simulink library "EmE_MBD_Blockset"  (R2018a)
settings: Solver=ode1  StartTime=0.0  StopTime=Inf  FixedStep=0.001  RelTol=1e-3  EnableMultiTasking=on
PostLoadFcn:
  | , if any(exist('dsrtsu_mdlpostloadfcn', 'file') == [2, 3, 6]), try dsrtsu_mdlpostloadfcn('Execute', bdroot); catch fprintf('Error in PostLoadFcn (dsrtsu_mdlpostloadfcn) for model "%s":\n %s\n', bdroot, lasterr); end, end,
undefined symbols (not defined in the file or in its folder): ENUM_TSC1_CONTROL_PURPOSE_T, gcbh, GLB_SWITCH_T
libraries: simulink x237, $bdroot x115, simulink_need_slupdate x26, MotoHawk_lib x13, simulink_extras x3
(part 2 of 11)

== system EmE_MBD_Blockset/Math Operators ==
  Abs : Abs  mask(Absolute value (EmE)){SaturateOnIntegerOverflow=off}
      mask prompts: SaturateOnIntegerOverflow "Simulink:blkprm_prompts:AllBlksSaturate"
      mask help: Outputs the absolute value of the input.
      mask TypeOptions SaturateOnIntegerOverflow: SaturateOnIntegerOverflow
      mask DialogControl SaturateOnIntegerOverflow Prompt: Saturate on integer overflow
  Add : Sum  InputSameDT=on
  Convert_polar_coordinates_to_rectangular_coordinates : Subsystem
  Convert_rectangular_coordinates_to_polar_coordinates : Subsystem
  Convert_time : Subsystem  mask(Convert units of time (EmE)){cvt_time_from=hr, cvt_time_to=min, sat_on_int_overflow=off}
      mask prompts: cvt_time_from "Convert time from"; cvt_time_to "Convert time to"; sat_on_int_overflow "Saturate on integer overflow"
      mask help:
      | Converts one unit of time to another.  Available time units are:
      | - microsecond (usec)
      | - millisecond (msec)
      | - second (sec)
      | - minute (min)
      | - hour (hr)
      | - day (day)
      | - year (yr)
      mask init:
      | constant = [get_param(gcbh,'Parent'),'/',get_param(gcbh,'name'),'/Constant'];
      | product1 = [get_param(gcbh,'Parent'),'/',get_param(gcbh,'name'),'/Product1'];
      | 
      | time_labels = ...
      |     { 'usec' 
      |       'msec' 
      |       'sec' 
      |       'min'
      |       'hr' 
      |       'day' 
      |       'yr' };
      | conversions_time = ...
      |     { '1'
      |       '1000'
      |       '1000'
      |       '60'
      |       '60'
      |       '24'
      |       '365'};
      | 
      | from_nr = find(strcmp(time_labels, cvt_time_from));
      | to_nr   = find(strcmp(time_labels, cvt_time_to));
      | 
      | conversion_factor = '1';
      | if ( from_nr < to_nr )
      |     for i = from_nr+1:to_nr
      |         conversion_factor = [conversion_factor, '/', conversions_time{i}];
      |     end
      | elseif ( from_nr > to_nr )
      |     for i = to_nr+1:from_nr
      |         conversion_factor = [conversion_factor, '*', conversions_time{i}];
      |     end
      | end
      | set_param(constant, 'Value', conversion_factor);
      | set_param(product1, 'SaturateOnIntegerOverflow', sat_on_int_overflow);
      mask TypeOptions cvt_time_from: usec | msec | sec | min | hr | day | yr
      mask TypeOptions cvt_time_to: usec | msec | sec | min | hr | day | yr
      mask Display: disp([cvt_time_from ' to ' cvt_time_to])
  Decrement Real World : simulink/Additional Math & Discrete/Additional Math: Increment - Decrement/Decrement Real World
      settings: SourceProductName=Simulink  SourceProductBaseCode=SL
  Divide : Product  Inputs=*/  InputSameDT=on
  Engineering_unit_conversion : Subsystem  mask(Convert engineering units (EmE)){eng_unit_type=torque, eng_unit_in=Nm, eng_unit_out=lbf-ft, sat_on_int_overflow=off}
      mask prompts: eng_unit_type "Unit type:"; eng_unit_in "Convert from:"; eng_unit_out "Convert to:"; sat_on_int_overflow "Saturate on integer overflow"
      mask help: Converts one engineering unit to another.
      mask init:
      | % https://www.mathworks.com/matlabcentral/fileexchange/3181-unit-conversion
      | unit_labels = {'accel','angle','area','density','energy','flow','flow_num','force','freq','fuel_econ','inertia','length','velocity','mass','power','pressure','spec_heat','temp','torque','kin_vis','vol'};
      | switch eng_unit_type,
      |     case 'accel',
      |         eng_unit_opts = {'cm/s2','ft/s2','g','m/s2','mi/hr-s','mm/s2'};
      |     case 'angle',
      |         eng_unit_opts = {'cycle','rad','deg','min','sec'};
      |     case 'area',
      |         eng_unit_opts = {'km2','hectare','m2','cm2','mm2','mile2','acre','ft2','in2'};
      |     case 'density',
      |         eng_unit_opts = {'tonne/m3','kg/m3','sg','lb/in3','lb/ft3','lb/igal','lb/usgal','slug/ft3'};
      |     case 'energy',
      |         eng_unit_opts = {'MJ','J','kWh','cal','chu','therm','btu','ft-lbf','hp-s'};
      |     case 'flow',
      |         eng_unit_opts = {'m3/s','liter/s','cc/s','in3/s','gal/hr','kg/s','lb/s','lb/hr','ft3/min'};
      |     case 'flow_num',
      |         eng_unit_opts = {'cc/s/sq(kPa)','ss/s/sq(bar)','gph/sq(psi)','in3/s/sq(psi)'};
      |     case 'force',
      |         eng_unit_opts = {'bar-m2','kN','N','kPa-mm2','dyne','kgf','tonf','lbf','pdl'};
      |     case 'freq',
      |         eng_unit_opts = {'1/ms','hz','rad/s','deg/s','rpm','1/hour','1/day'};
      |     case 'fuel_econ',
      |         eng_unit_opts = {'100km/l','km/l','m/l','mi/igal','mi/usgal'};
      |     case 'inertia',
      |         eng_unit_opts = {'kg-m2','lb-ft2','lb-in2'};
      |     case 'length',
      |         eng_unit_opts = {'km','m','cm','mm','n-mile','mile','yard','ft','in'};
      |     case 'velocity',
      |         eng_unit_opts = {'km/s','km/hr','m/s','m/min','m/hr','knot','mph','ft/s','ft/hr'};
      |     case 'mass',
      |         eng_unit_opts = {'tonne','kg','g','ton','slug','stone','lb','oz','dr'};
      |     case 'power',
      |         eng_unit_opts = {'kw','w','chu/s','btu/s','btu/hr','ft-lbf/s','ps','hp'};
      |     case 'pressure',
      |         eng_unit_opts = {'MPa','bar','kPa','Pa','atm','ton/in2','psi','mmHg'};
      |     case 'spec_heat',
      |         eng_unit_opts = {'kJ/kg-K','J/kg-K','chu/lb-K','btu/lb-R','hp-s/lb-K','ft-lbf/lb-R'};
      |     case 'temp',
      |         eng_unit_opts = {'K','C','R','F'};
      |     case 'torque',
      |         eng_unit_opts = {'Nm','lbf-ft','lbf-in'};
      |     case 'kin_vis',
      |         eng_unit_opts = {'m2/s','cm2/s','cStoke','ft2/s','in2/s'};
      |     case 'vol',
      |         eng_unit_opts = {'m3','liter','cm3','mm3','ft3','in3','igal','pint','usgal'};
      | end;
      | % set table parameters
      | unit_type_idx = [];
      | unit_in_type_idx = [];
      | unit_out_type_idx = [];
      | user_sg=1; % specific gravity value used... need to add to dialog?
      | try
      |     unit_type_idx = find(strcmpi(unit_labels, eng_unit_type));
      |     unit_in_type_idx = find(strcmpi(eng_unit_opts, eng_unit_in));
      |     unit_out_type_idx = find(strcmpi(eng_unit_opts, eng_unit_out));
      | catch
      | end;
      | if (~isempty(unit_type_idx) && ~isempty(unit_in_type_idx) && ~isempty(unit_out_type_idx)),
      |     % Set output size
      |     opsiz=[1,1];
      |     oplen=prod(opsiz);
      |     
      |     % Define basic numbers
      |     yd=1/0.9144; yd2=yd^2; yd3=yd*yd2; mi=1760; acr=4840; gal=1/4.546092; usgl=231;
      |     lb=1/0.45359237; ton=2240; g=9.80665; atm=101.325; hg=750.0616827e-5;
      |     ps=1/75; hp=550; cal=0.238846; chu=1/1899.1005354; k2r=1.8; abz=273.15;
      |     sg=1;
      |     
      |     % For future development - if required
      |     % angstrom=1e-10m; rod=5.5yard; chain=22yard; furlong=10chain; fathom=2yard;
      |     % short_ton=2000 lb; cwt=112 lb; lb=7000grain; metric_carat=0.2g;
      |     % chaldron=36bushel; barrel=36gal bushel=8gal; peck=2gal; quart=2pint; pint=4gill; gill=5fl.oz; fl.oz=8fl.drachm
      |     
      |     fact = [...
      |         1,0.0328083,0.0010197,0.01,0.0223692,10,0,0,0;...                                               % accel
      |         1/2,pi,180,180*60,180*3600,0,0,0,0;...                                                          % angle
      |         1e-6,1e-4,1,1e4,1e6,yd2/mi^2,yd2/acr,9*yd2,1296*yd2;...                                         % area
      |         1e-3,1,1e-3,lb/(46656*yd3),lb/(27*yd3),lb/(1e3*gal),lb*usgl/(46656*yd3),lb/(81*yd2^2*g),0;...   % density
      |         1e-6,1,1e-6/3.6,cal,chu,chu*k2r*1e-5,chu*k2r,3*yd*lb/g,3*yd*lb/g/hp;...                         % energy
      |         1e-6,1e-3,1,0.046656*yd3,gal*3.6,sg*1e-3,lb*sg*1e-3,lb*sg*1e-1*36,0.00211888;...                % flow
      |         1,10,gal*yd*12.96*sqrt(0.1*g/lb),(0.1296*yd2)^2*sqrt(10*g/lb),0,0,0,0,0;...                     % flow_num
      |         1e-5,1e-3,1,1e3,1e5,1/g,lb/(g*ton),lb/g,lb*yd*3;...                                             % force
      |         1e-3,1,2*pi,360,60,3600,86400,0,0;...                                                           % freq
      |         1e-5,1e-3,1,yd/(mi*gal),yd*usgl/(mi*yd3*46.656),0,0,0,0;...                                     % fuel_econ
      |         1,lb*9*yd2,lb*1296*yd2,0,0,0,0,0,0;...                                                          % inertia
      |         1e-3,1,100,1000,1/1852,yd/mi,yd,3*yd,36*yd;...                                                  % length
      |         1e-3,3.6,1,60,3600,3600/1852,yd*3600/mi,3*yd,3*yd*3600;...                                      % velocity
      |         1e-3,1,1000,lb/ton,lb/(yd*3*g),lb/14,lb,lb*16,lb*16^2;...                                       % mass
      |         1e-3,1,chu,chu*k2r,chu*k2r*3600,3*yd*lb/g,ps/g,3*yd*lb/g/hp,0;...                               % power
      |         1e-6,1e-5,1e-3,1,1e-3/atm,lb/(1296*ton*g*yd2),lb/(1296*g*yd2),hg,0;...                          % pressure
      |         1e-3,1,chu/lb,chu/lb,3*yd/(g*hp),3*yd/g/k2r,0,0,0;...                                           % spec_heat
      |         1,1,k2r,k2r,0,0,0,0,0;...                                                                       % temp
      |         1,0.737561,8.85075,0,0,0,0,0,0;...                                                              % torque
      |         1,1e4,1e6,9*yd2,1296*yd2,0,0,0,0;...                                                            % kin_vis
      |         1,1e3,1e6,1e9,27*yd3,27*yd3*1728,1e3*gal,gal*8000,yd3*46656/usgl;...                            % vol
      |         ];
      |     off = [abz,0,abz,32/k2r,0,0,0,0,0];                                                                 % temp
      |     
      |     % Set factor
      |     % sub2ind indexes into a matrix; matrix(a,b) is a matrix if both a & b are vectors
      |     ind=sub2ind( size(fact), ones(oplen,1).*unit_type_idx(:), ones(oplen,1).*unit_in_type_idx(:) );
      |     in_fact=fact(ind);
      |     ind=sub2ind( size(fact), ones(oplen,1).*unit_type_idx(:), ones(oplen,1).*unit_out_type_idx(:) );
      |     out_fact=fact(ind);
      |     
      |     % Set offset - apply if unit_type_idx==18(temp), else 0
      |     in_off=off(unit_in_type_idx(:))'.*(unit_type_idx(:)==18);
      |     out_off=off(unit_out_type_idx(:))'.*(unit_type_idx(:)==18);
      |     
      |     % Previous un-vectorised code:-
      |     % If user chose Qflow & Mflow use sg - sg defaults 1, keep here in case it's changed
      |     %if unit_type_idx==5 & ((unitinput>5) ~= (unitoutput>5))
      |     %  if unitinput>5 then
      |     %     in_fact = in_fact(:) .* user_sg(:)/sg;
      |     %  else
      |     %     out_fact = out_fact(:) .* user_sg(:)/sg;
      |     %  end;
      |     %end;
      |     % This sg thing adds a complication for vector/matrix arithmetic:
      |     flow_conv=(unit_type_idx(:)==6 & ((unit_in_type_idx(:)>6) ~= (unit_out_type_idx(:)>6))); % vector of whether sg is needed
      |     ip_gt_6=(unit_in_type_idx(:)>6)*2-1;  % vector of 1 or -1 s : 1->multiply; (-1)->divide
      |     in_fact = in_fact(:) .* ((user_sg(:)/sg) .^ flow_conv).^ip_gt_6;
      |     
      |     % Set factor & offset
      |     factor_u=out_fact(:)./in_fact(:);
      |     offset_u=(out_off(:)-in_off(:)).*out_fact(:);
      |     
      |     % Reshape to match unitinput matrix size
      |     factor_u=reshape(factor_u,opsiz);
      |     offset_u=reshape(offset_u,opsiz);
      | end;
      | % assign values in simulink block
      | gain_value = [get_param(gcbh,'Parent'),'/',get_param(gcbh,'name'),'/Gain_value'];
      | offset_value = [get_param(gcbh,'Parent'),'/',get_param(gcbh,'name'),'/Offset_value'];
      | set_param(gain_value, 'Value', num2str(factor_u));
      | set_param(offset_value, 'Value', num2str(offset_u));
      mask TypeOptions eng_unit_type: accel | angle | area | density | energy | flow | flow_num | force | freq | fuel_econ | inertia | length | velocity | mass | power | pressure | spec_heat | temp | torque | kin_vis | vol
      mask Callback eng_unit_type:
      | % https://www.mathworks.com/matlabcentral/answers/82930-dynamically-populating-mask-parameter-popup-list
      | % get the unit type selected
      | eng_unit_type_gcbh = get(gcbh);
      | eng_unit_type = eng_unit_type_gcbh.eng_unit_type;
      | % begin to set the 'from' and 'to' unit type drop down menus
      | maskstyles = get_param(gcb, 'MaskStyles');
      | switch eng_unit_type,
      |     case 'accel',
      |         eng_unit_opts = 'popup(cm/s2|ft/s2|g|m/s2|mi/hr-s|mm/s2)';
      |     case 'angle',
      |         eng_unit_opts = 'popup(cycle|rad|deg|min|sec)';
      |     case 'area',
      |         eng_unit_opts = 'popup(km2|hectare|m2|cm2|mm2|mile2|acre|ft2|in2)';
      |     case 'density',
      |         eng_unit_opts = 'popup(tonne/m3|kg/m3|sg|lb/in3|lb/ft3|lb/igal|lb/usgal|slug/ft3)';
      |     case 'energy',
      |         eng_unit_opts = 'popup(MJ|J|kWh|cal|chu|therm|btu|ft-lbf|hp-s)';
      |     case 'flow',
      |         eng_unit_opts = 'popup(m3/s|liter/s|cc/s|in3/s|gal/hr|kg/s|lb/s|lb/hr|ft3/min)';
      |     case 'flow_num',
      |         eng_unit_opts = 'popup(cc/s/sq(kPa)|ss/s/sq(bar)|gph/sq(psi)|in3/s/sq(psi))';
      |     case 'force',
      |         eng_unit_opts = 'popup(bar-m2|kN|N|kPa-mm2|dyne|kgf|tonf|lbf|pdl)';
      |     case 'freq',
      |         eng_unit_opts = 'popup(1/ms|hz|rad/s|deg/s|rpm|1/hour|1/day)';
      |     case 'fuel_econ',
      |         eng_unit_opts = 'popup(100km/l|km/l|m/l|mi/igal|mi/usgal)';
      |     case 'inertia',
      |         eng_unit_opts = 'popup(kg-m2|lb-ft2|lb-in2)';
      |     case 'length',
      |         eng_unit_opts = 'popup(km|m|cm|mm|n-mile|mile|yard|ft|in)';
      |     case 'velocity',
      |         eng_unit_opts = 'popup(km/s|km/hr|m/s|m/min|m/hr|knot|mph|ft/s|ft/hr)';
      |     case 'mass',
      |         eng_unit_opts = 'popup(tonne|kg|g|ton|slug|stone|lb|oz|dr)';
      |     case 'power',
      |         eng_unit_opts = 'popup(kw|w|chu/s|btu/s|btu/hr|ft-lbf/s|ps|hp)';
      |     case 'pressure',
      |         eng_unit_opts = 'popup(MPa|bar|kPa|Pa|atm|ton/in2|psi|mmHg)';
      |     case 'spec_heat',
      |         eng_unit_opts = 'popup(kJ/kg-K|J/kg-K|chu/lb-K|btu/lb-R|hp-s/lb-K|ft-lbf/lb-R)';
      |     case 'temp',
      |         eng_unit_opts = 'popup(K|C|R|F)';
      |     case 'torque',
      |         eng_unit_opts = 'popup(Nm|lbf-ft|lbf-in)';
      |     case 'kin_vis',
      |         eng_unit_opts = 'popup(m2/s|cm2/s|cStoke|ft2/s|in2/s)';
      |     case 'vol',
      |         eng_unit_opts = 'popup(m3|liter|cm3|mm3|ft3|in3|igal|pint|usgal)';
      | end;
      | 
      | % set the other drop down menu boxes with the selectable units
      | maskstyles{2} = eng_unit_opts;
      | maskstyles{3} = eng_unit_opts;
      | set_param(gcb, 'MaskStyles', maskstyles);
      mask TypeOptions eng_unit_in: Nm | lbf-ft | lbf-in
      mask TypeOptions eng_unit_out: Nm | lbf-ft | lbf-in
      mask Display:
      | % sprintf('%s/n%s to %s',[engunittype,engunitinput,engunitoutput])
      | disp([eng_unit_type '\n' eng_unit_in ' to ' eng_unit_out])
  Find Nonzero Elements : Find  NumberOfInputDimensions=3  IndexMode=Zero-based
  Gain : Gain
  Generic_linear_function : Subsystem  mask(Generic linear function (EmE)){}
      mask help: Linear interpolation function for x-y interpolation. Output is bound by Y1 and Y2 values.
      mask init:
      | X_1=0.37;
      | X_2=0.65;
      | Y_1=0.37;
      | Y_2=0.8;
      mask Display:
      | %AXIS
      |     plot([0.2 0.8]+0.15,[0.3 0.3]+0.1);
      |     plot([0.25 0.25]+0.15,[0.25 0.97]+0.1);
      |     text(0.38,1.05,'y')
      |     text(0.93,0.39,'x')
      | 
      | % GRAPH
      |     plot([X_1 X_2]+0.15,[Y_1 Y_2]+0.1)
      | 
      | % TEXT and LINES
      | %X_1
      |     plot([X_1,X_1]+0.15,[0.37 0.36]+0.1);
      |     plot([X_1,X_1]+0.15,[0.34 0.33]+0.07);
      |     plot([X_1,X_1]+0.15,[0.33 0.31]+0.1);
      |     text(0.49,0.33,sprintf('%s\n','X1'))
      | 
      | %X_2
      |     plot([Y_1 Y_1]+0.43,[0.25 0.28]+0.61);
      |     plot([Y_1 Y_1]+0.43,[0.22 0.19]+0.61);
      |     plot([Y_1 Y_1]+0.43,[0.16 0.13]+0.61);
      |     plot([Y_1 Y_1]+0.43,[0.10 0.07]+0.61);
      |     plot([Y_1 Y_1]+0.43,[0.04 0.01]+0.61);
      |     plot([Y_1 Y_1]+0.43,[-0.02 -0.05]+0.61);
      |     plot([Y_1 Y_1]+0.43,[-0.08 -0.11]+0.61);
      |     plot([Y_1 Y_1]+0.43,[-0.14 -0.17]+0.61);
      |     plot([Y_1 Y_1]+0.43,[-0.20 -0.21]+0.61);
      |     text(0.77,0.33,sprintf('%s\n','X2'))
      | 
      | %Y_1
      |     plot([0.3 0.42]+0.1,[Y_1 Y_1]+0.1);
      |     text(0.3,0.48,'Y1')
      | 
      | %Y_2
      |     plot([0.25 0.28]+0.15,[X_2 X_2]+0.25);
      |     plot([0.31 0.34]+0.15,[X_2 X_2]+0.25);
      |     plot([0.37 0.40]+0.15,[X_2 X_2]+0.25);
      |     plot([0.43 0.46]+0.15,[X_2 X_2]+0.25);
      |     plot([0.49 0.52]+0.15,[X_2 X_2]+0.25);
      |     plot([0.55 0.58]+0.15,[X_2 X_2]+0.25);
      |     plot([0.61 0.64]+0.15,[X_2 X_2]+0.25);
      |     plot([0.65 0.8]+0.15,[X_2 X_2]+0.25);
      |     text(0.3,Y_2+0.1,'Y2')
      | 
      | %Center pic
      | text(0.16,1.3,' ')
      | text(1.1,0.1,' ')
  Increment Real World : simulink/Additional Math & Discrete/Additional Math: Increment - Decrement/Increment Real World
      settings: SourceProductName=Simulink  SourceProductBaseCode=SL
  Math Function : Math  SaturateOnIntegerOverflow=on
  MinMax : MinMax  Inputs=2  InputSameDT=on
  MinMax Running Resettable : simulink/Math Operations/MinMax Running Resettable  Function=min  vinit=0
      settings: AttributesFormatString=IC: %<vinit>
  Min_max_index : Subsystem  mask(Min max index (EmE)){func=max, sat_on_int_overflow=off}
      mask prompts: func "Function:"; sat_on_int_overflow "Saturate on integer overflow"
      mask help:
      | Output min or max of the inputs as well as the index of the winning input.  The inputs are prioritized from top to bottom.
      | Input to the block must be a bus or a mux.
      mask init:
      | minmaxblk = [get_param(gcbh,'parent'),'/',get_param(gcbh,'name'),'/MinMax'];
      | set_param(minmaxblk,'Function',func);
      mask TypeOptions func: min | max
      mask Display:
      | disp(func);
      | port_label('output', 1, 'v');
      | port_label('output', 2, 'i');
  Normalize_on_min_max : Subsystem  mask(Normalize on min, max (EmE)){sel=Min}
      mask prompts: sel "Normalize on:"
      mask help: Normalize the input on the minimum or maximum boundary.
      mask init:
      | cpv = [get_param(gcbh,'parent'),'/',get_param(gcbh,'name'),'/Constant'];
      | if strcmp(sel,'Min'),
      |     set_param(cpv,'Value','true');
      | else,
      |     set_param(cpv,'Value','false');
      | end
      mask TypeOptions sel: Min | Max
      mask Display:
      | plot([0.1 0.1 0.8 0.8],[0.3 0.7 0.7 0.3])
      | plot([0.1 0.8],[0.3 0.3])
      | text( 0.15, 0.5, 'norm =')
      | plot([0.4 0.75],[0.5 0.5])
      | text( 0.43, 0.4, '(max - min)')
      | if (strcmpi(sel,'Min')),
      |     text( 0.45, 0.6, '(in - min)')
      | else,
      |     text( 0.45, 0.6, '(max - in)')
      | end;
  Product : Product  InputSameDT=on
  Rounding Function : Rounding  mask(Rounding function (EmE)){Operator=floor}
      mask prompts: Operator "Simulink:blkprm_prompts:RoundOperator"
      mask help: Apply rounding function to signal.
      mask TypeOptions Operator: Operator
      mask DialogControl Operator Prompt: Function:
  Slew : Subsystem  mask(Slew (EmE)){}
      mask help:
      | Limits the maximum increase rate by 'Inc' and the maximum decrease rate by 'Dec'.
      | If In > Out, then Out is increased by Inc*dT every time step until Out = In.
      | If In < Out, then Out is decreased by Dec*dT every time step until Out = In.
      mask Display:
      | plot([0.1 1],[0.5 0.96])
      | plot([0.1 1],[0.5 0.04])
      | plot([0.1 0.7],[0.5 0.5])
      | plot([0.65 0.7],[0.55 0.5])
      | plot([0.65 0.7],[0.45 0.5])
      | 
      | plot([0 0.22],[0.8 0.58])
      | plot([0 0.22],[0.2 0.42])
      | plot([0.1 0.42],[1 0.68])
      | plot([0.1 0.42],[0 0.32])
      | plot([0.4 0.62],[1 0.78])
      | plot([0.4 0.62],[0 0.22])
      | plot([0.7 0.81],[1 0.88])
      | plot([0.7 0.81],[0 0.12])
  Slew_at_event : Subsystem  mask(Slew at event (EmE)){}
      mask help:
      | Performs a trigger-based slew that is initialized with value Init and slews towards In at a linear rate defined by Inc and Dec.
      | dT defines the sample time of the block.
      | F_Out_slewing is TRUE if the absolute difference between In and Out is >1 and F_Event_trigger was TRUE for at least one cycle.
      mask Display:
      | % the trigger input graphic
      | plot([0.2 0.3 0.3 0.35 0.35 0.6],[0.7 0.7 0.8 0.8 0.7 0.7])
      | plot([0.6 0.6 0.6 0.65 0.65 0.8],[0.7 0.7 0.8 0.8 0.7 0.7])
      | text(0.25, 0.65, 'trigger')
      | 
      | % the output value graphic
      | plot([0.2 0.3 0.4 0.6 0.7 0.8],[0.25 0.25 0.55 0.55 0.25 0.25])
      | text(0.25, 0.2, 'out')
  Slew_init_reset : Subsystem  mask(Slew init reset (EmE)){}
      mask help:
      | Limits the maximum increase rate by 'Inc' and the maximum decrease rate by 'Dec'.
      | Can be reset to a custom initial value (Init).
      | If In > Out, then Out is increased by Inc*dT every time step until Out = In.
      | If In < Out, then Out is decreased by Dec*dT every time step until Out = In.
      mask Display:
      | plot([0.1 1],[0.5 0.96])
      | plot([0.1 1],[0.5 0.04])
      | plot([0.1 0.7],[0.5 0.5])
      | plot([0.65 0.7],[0.55 0.5])
      | plot([0.65 0.7],[0.45 0.5])
      | 
      | plot([0 0.22],[0.8 0.58])
      | plot([0 0.22],[0.2 0.42])
      | plot([0.1 0.42],[1 0.68])
      | plot([0.1 0.42],[0 0.32])
      | plot([0.4 0.62],[1 0.78])
      | plot([0.4 0.62],[0 0.22])
      | plot([0.7 0.81],[1 0.88])
      | plot([0.7 0.81],[0 0.12])
  Slope_intercept : Subsystem  mask(Slope intercept){}
      mask help:
      | Determines the slope intercept values (or linear equation): y=mx+b,
      | where m is the gain and b is the offset.
      mask Display:
      | text(0.25, 0.65, 'm=(y2-y1)/(x2-x1)')
      | text(0.25, 0.45, 'b=(y1-(x1*m)')
  Soft_transition : Subsystem  mask(Soft transition (EmE)){}
      mask help:
      | Output is slewed from Input value changes.
      | Output will equal Input at T_Inc seconds upon rising changes in Input.
      | Output will equal Input at T_Dec seconds upon falling changes in Input.
      | dT is determined internally.
      mask Display: plot([0.2 0.3 0.4 0.6 0.7 0.8],[0.25 0.25 0.75 0.75 0.25 0.25])
  Subtract : Sum  Inputs=+-  InputSameDT=on

== system EmE_MBD_Blockset/Obsolete ==
  Normalize_on_max : Subsystem  mask(Normalize on max (EmE)){}
      mask help: Normalize the input on the maximum boundary.
      mask Display:
      | plot([0.1 0.1 0.8 0.8],[0.3 0.7 0.7 0.3])
      | plot([0.1 0.8],[0.3 0.3])
      | text( 0.15, 0.5, 'norm =')
      | text( 0.45, 0.6, '(max - in)')
      | plot([0.4 0.75],[0.5 0.5])
      | text( 0.43, 0.4, '(max - min)')
  Normalize_on_min : Subsystem  mask(Normalize on min (EmE)){}
      mask help: Normalize the input on the minimum boundary.
      mask Display:
      | plot([0.1 0.1 0.8 0.8],[0.3 0.7 0.7 0.3])
      | plot([0.1 0.8],[0.3 0.3])
      | text( 0.15, 0.5, 'norm =')
      | text( 0.45, 0.6, '(in - min)')
      | plot([0.4 0.75],[0.5 0.5])
      | text( 0.43, 0.4, '(max - min)')

== system EmE_MBD_Blockset/Ports and Subsystems ==
  In : Inport
  Enable : EnablePort  StatesWhenEnabling=reset
      settings: AttributesFormatString=States when enabling: %<StatesWhenEnabling>
      settings: CopyFcn=|
      | try
      | L = find_system(get(gcbh,'Parent'),'BlockType','Outport');
      | M = find_system(get(gcbh,'Parent'),'BlockType','EnablePort');
      | N = find_system(get(gcbh,'Parent'),'BlockType','TriggerPort');
      | anyoutports = ~isempty(L);
      | anyenableports = ~isempty(M);
      | anytriggerports = ~isempty(N);
      | sys = get_param(L,'Handle');
      | noutports = length(sys);
      | if (anyoutports),
      | for i = 1:noutports,
      | set(sys{i},'AttributesFormatString','IC: %<InitialOutput>\nDisabled value: %<OutputWhenDisabled>')
      | end;
      | end;
      | catch
      | end;
      | clear i L M N anyoutports anyenableports anytriggerports sys noutports
      settings: DeleteFcn=|
      | try
      | L = find_system(get(gcbh,'Parent'),'BlockType','Outport');
      | M = find_system(get(gcbh,'Parent'),'BlockType','EnablePort');
      | N = find_system(get(gcbh,'Parent'),'BlockType','TriggerPort');
      | anyoutports = ~isempty(L);
      | anyenableports = ~isempty(M);
      | anytriggerports = ~isempty(N);
      | sys = get_param(L,'Handle');
      | noutports = length(sys);
      | if ((anyoutports) && (~anytriggerports)),
      | for i = 1:noutports,
      | set(sys{i},'AttributesFormatString','')
      | end;
      | end;
      | catch
      | end;
      | clear i L M N anyoutports anyenableports anytriggerports sys noutports
      settings: NameChangeFcn=|
      | try
      | L = find_system(get(gcbh,'Parent'),'BlockType','Outport');
      | M = find_system(get(gcbh,'Parent'),'BlockType','EnablePort');
      | N = find_system(get(gcbh,'Parent'),'BlockType','TriggerPort');
      | anyoutports = ~isempty(L);
      | anyenableports = ~isempty(M);
      | anytriggerports = ~isempty(N);
      | sys = get_param(L,'Handle');
      | noutports = length(sys);
      | if (anyoutports),
      | for i = 1:noutports,
      | set(sys{i},'AttributesFormatString','IC: %<InitialOutput>\nDisabled value: %<OutputWhenDisabled>')
      | end;
      | end;
      | catch
      | end
      | clear i L M N anyoutports anyenableports anytriggerports sys noutports
      settings: MoveFcn=|
      | try
      | L = find_system(get(gcbh,'Parent'),'BlockType','Outport');
      | M = find_system(get(gcbh,'Parent'),'BlockType','EnablePort');
      | N = find_system(get(gcbh,'Parent'),'BlockType','TriggerPort');
      | anyoutports = ~isempty(L);
      | anyenableports = ~isempty(M);
      | anytriggerports = ~isempty(N);
      | sys = get_param(L,'Handle');
      | noutports = length(sys);
      | if (anyoutports),
      | for i = 1:noutports,
      | set(sys{i},'AttributesFormatString','IC: %<InitialOutput>\nDisabled value: %<OutputWhenDisabled>')
      | end;
      | end;
      | catch
      | end;
      | clear i L M N anyoutports anyenableports anytriggerports sys noutports
  Trigger : TriggerPort  VariantControl=(inherit)
      settings: AttributesFormatString=States when enabling: %<StatesWhenEnabling>
      settings: CopyFcn=|
      | try
      | L = find_system(get(gcbh,'Parent'),'BlockType','Outport');
      | M = find_system(get(gcbh,'Parent'),'BlockType','EnablePort');
      | N = find_system(get(gcbh,'Parent'),'BlockType','TriggerPort');
      | anyoutports = ~isempty(L);
      | anyenableports = ~isempty(M);
      | anytriggerports = ~isempty(N);
      | sys = get_param(L,'Handle');
      | noutports = length(sys);
      | if (anyoutports),
      | for i = 1:noutports,
      | set(sys{i},'AttributesFormatString','IC: %<InitialOutput>\nDisabled value: %<OutputWhenDisabled>')
      | end;
      | end;
      | catch
      | end;
      | clear i L M N anyoutports anyenableports anytriggerports sys noutports
      settings: DeleteFcn=|
      | try
      | L = find_system(get(gcbh,'Parent'),'BlockType','Outport');
      | M = find_system(get(gcbh,'Parent'),'BlockType','EnablePort');
      | N = find_system(get(gcbh,'Parent'),'BlockType','TriggerPort');
      | anyoutports = ~isempty(L);
      | anyenableports = ~isempty(M);
      | anytriggerports = ~isempty(N);
      | sys = get_param(L,'Handle');
      | noutports = length(sys);
      | if ((anyoutports) && (~anyenableports)),
      | for i = 1:noutports,
      | set(sys{i},'AttributesFormatString','')
      | end;
      | end;
      | catch
      | end;
      | clear i L M N anyoutports anyenableports anytriggerports sys noutports
      settings: NameChangeFcn=|
      | try
      | L = find_system(get(gcbh,'Parent'),'BlockType','Outport');
      | M = find_system(get(gcbh,'Parent'),'BlockType','EnablePort');
      | N = find_system(get(gcbh,'Parent'),'BlockType','TriggerPort');
      | anyoutports = ~isempty(L);
      | anyenableports = ~isempty(M);
      | anytriggerports = ~isempty(N);
      | sys = get_param(L,'Handle');
      | noutports = length(sys);
      | if (anyoutports),
      | for i = 1:noutports,
      | set(sys{i},'AttributesFormatString','IC: %<InitialOutput>\nDisabled value: %<OutputWhenDisabled>')
      | end;
      | end;
      | catch
      | end;
      | clear i L M N anyoutports anyenableports anytriggerports sys noutports
      settings: MoveFcn=|
      | try
      | L = find_system(get(gcbh,'Parent'),'BlockType','Outport');
      | M = find_system(get(gcbh,'Parent'),'BlockType','EnablePort');
      | N = find_system(get(gcbh,'Parent'),'BlockType','TriggerPort');
      | anyoutports = ~isempty(L);
      | anyenableports = ~isempty(M);
      | anytriggerports = ~isempty(N);
      | sys = get_param(L,'Handle');
      | noutports = length(sys);
      | if (anyoutports),
      | for i = 1:noutports,
      | set(sys{i},'AttributesFormatString','IC: %<InitialOutput>\nDisabled value: %<OutputWhenDisabled>')
      | end;
      | end;
      | catch
      | end;
      | clear i L M N anyoutports anyenableports anytriggerports sys noutports
  Enabled Subsystem : Subsystem  LoadFcn=set_param(gcbh,'LinkStatus','none')  ClipboardFcn=set_param(gcbh,'LinkStatus','none')  TreatAsAtomicUnit=on
      settings: CopyFcn=set_param(gcbh,'LinkStatus','none')  NameChangeFcn=set_param(gcbh,'LinkStatus','none')  MoveFcn=set_param(gcbh,'LinkStatus','none')
  Enabled and Triggered Subsystem : Subsystem  LoadFcn=set_param(gcbh,'LinkStatus','none')  ClipboardFcn=set_param(gcbh,'LinkStatus','none')  TreatAsAtomicUnit=on
      settings: CopyFcn=set_param(gcbh,'LinkStatus','none')  NameChangeFcn=set_param(gcbh,'LinkStatus','none')  MoveFcn=set_param(gcbh,'LinkStatus','none')
  Subsystem : Subsystem  LoadFcn=set_param(gcbh,'LinkStatus','none')  ClipboardFcn=set_param(gcbh,'LinkStatus','none')
      settings: CopyFcn=set_param(gcbh,'LinkStatus','none')  NameChangeFcn=set_param(gcbh,'LinkStatus','none')  MoveFcn=set_param(gcbh,'LinkStatus','none')
  Triggered Subsystem : Subsystem  LoadFcn=set_param(gcbh,'LinkStatus','none')  ClipboardFcn=set_param(gcbh,'LinkStatus','none')  TreatAsAtomicUnit=on
      settings: CopyFcn=set_param(gcbh,'LinkStatus','none')  NameChangeFcn=set_param(gcbh,'LinkStatus','none')  MoveFcn=set_param(gcbh,'LinkStatus','none')
  Out : Outport  LibraryBlock=$bdroot/Sinks/Out  OutputWhenDisabled=reset
      settings: AttributesFormatString=IC: %<InitialOutput>\nDisabled value: %<OutputWhenDisabled>

== system EmE_MBD_Blockset/Signal Attributes ==
  Data Type Conversion : DataTypeConversion  mask(Data type conversion (EmE)){OutDataTypeStr=Inherit: Inherit via back propagation, SaturateOnIntegerOverflow=off}
      mask prompts: OutDataTypeStr "Simulink:blkprm_prompts:OUTPUT_UNIFIEDDATATYPE"; SaturateOnIntegerOverflow "Simulink:blkprm_prompts:AllBlksSaturate"
      mask help: Convert from one data type to another.
      mask init:
      | a = get(gcbh);
      | b = a.OutDataTypeStr;
      | if(any(strfind(b,'Enum: '))),
      | set(gcbh,'AttributesFormatString','%<OutDataTypeStr>');
      | else
      | set(gcbh,'AttributesFormatString','');
      | end;
      mask TypeOptions OutDataTypeStr: OutDataTypeStr
      mask TypeOptions SaturateOnIntegerOverflow: SaturateOnIntegerOverflow

== system EmE_MBD_Blockset/Signal Routing ==
  Bus Creator : BusCreator  Inputs=2
  Bus Selector : BusSelector  OutputSignals=signal1,signal2
  Demux : Demux  Outputs=2
  Enumerated Switch : MultiPortSwitch  DataPortOrder=Specify indices  Inputs=6  DataPortIndices=DataPortIndices  DataPortForDefault=Additional data port  DiagnosticForDefault=None  InputSameDT=on  mask(Enumeration switch (EmE)){enum_class=GLB_SWITCH_T, sel_indices=All, DataPortIndices={GLB_SWITCH_T.OFF,GLB_SWITCH_T.ON,GLB_SWITCH_T.ERROR,GLB_SWITCH_T.NOT_AVAILABLE}, fpath=C:\data\svn\PowerTrainSys\trunk\src\Projects_RCP\MY2017_RCP\EmE_MBD_Blockset\GLB_SWITCH_T.m}
      mask prompts: enum_class "Enumeration:"; sel_indices "Values"; DataPortIndices "Simulink:blkprm_prompts:MpSwitch_DataPortIndices"; fpath "Source:"
      mask help: Choose between multiple block inputs based on an enumerated signal.
      mask init:
      | cbid = get(gcbh); % get current block handle (in this case, is the mask)
      | cbvalues = cbid.MaskValues; % get the values from the mask
      | cbenables = cbid.MaskEnables; % get the enables from the mask
      | % enum_class = char(cbvalues(1)); % enum name
      | [fpathstr,fnamestr,fextstr]=fileparts(char(cbvalues(4)));
      | enum_class = fnamestr; % enum name
      | cbvalues(1) = cellstr(fnamestr);
      | set(gcbh,'MaskValues',cbvalues);
      | % % enum_location = which(enum_class) % enum file path
      | % % [fpathstr,fname,fext] = fileparts(enum_location);
      | % % enum_location = enum_location(1,:); % to prevent shadowed files
      | % % fileexists = 0;
      | % % try
      | % %     if (exist(enum_location) == 2), fileexists = 1; end;
      | % % catch
      | % % end;
      | % % if (fileexists),
      | % %     cbvalues(1) = cellstr(fname);
      | % %     cbvalues(4) = cellstr(enum_location);
      | % %     set(gcbh,'MaskValues',cbvalues);
      | % % end;
      | % 
      | % if (ismember('All',cbvalues(2))), % if radio button selection (MaskValues = 2) is 'All'
      | %     cbenables(3) = {'off'}; % disable the edit box
      | %     tenum_class = cbvalues(1); % assign value of enum name in textbox to variable
      | %     enum_values = enumeration(tenum_class{1}); % get enumeration values based on enum name in textbox
      | %     nenums = length(enum_values); % # of enumeration values
      | %     possible_enums = ['{' char(tenum_class) '.'];
      | %     % get enum values and make cell
      | %     for i = 1:nenums,
      | %         thisenum = char(enum_values(i));
      | %         if (i == 1),
      | %             possible_enums = strcat(possible_enums,thisenum);
      | %         else
      | %             possible_enums = strcat(possible_enums,',',tenum_class,'.',thisenum);
      | %         end;
      | %     end;
      | %     possible_enums = char(strcat(possible_enums,'}'));
      | %     set(gcbh,'DataPortIndices',possible_enums);
      | %     cbvalues(3) = cellstr(possible_enums);
      | %     set(gcbh,'MaskValues',cbvalues);
      | % %     % populate the edit box with all of the possible enumeration values
      | % %     enum_values = cbvalues(1); % assign value of enum name in textbox to variable
      | % %     enum_values = enumeration(enum_values{1}); % get enumeration values based on enum name in textbox
      | % %     nenums = length(enum_values); % # of enumeration values
      | % %     % get enum values and make cell
      | % %     for i = 1:nenums, % create enum value string separated by commas
      | % %         thisenum = char(enum_values(i));
      | % %         if (i == 1),
      | % %             possible_enums = ['{''' thisenum ''''];
      | % %             dataportindices_enums = ['{' enum_class '.' thisenum];
      | % %         else
      | % %             possible_enums = [possible_enums ',''' thisenum ''''];
      | % %             dataportindices_enums = [dataportindices_enums ',' enum_class '.' thisenum];
      | % %         end;
      | % %     end;
      | % %     possible_enums = [possible_enums '}']; % displayed enum
      | % %     dataportindices_enums = [dataportindices_enums '}']; % actual enum values
      | % %     set(gcbh,'DataPortIndices',dataportindices_enums); % set actual enum values
      | % %     possible_enums = cellstr(possible_enums); % set displayed enum values as cell
      | % %     cbvalues(3) = possible_enums; % store displayed enum values
      | % %     set(gcbh,'MaskValues',cbvalues); % store displayed enum values
      | % else % if radio button selection (MaskValues = 2) is NOT 'All'; custom block setup
      | %     cbenables(3) = {'on'}; % enable the edit box
      | % %     enums = cbvalues(3) % raw text from textbox
      | % %     separatorpos = strfind(enums,',') % find all commas, enums must be separated by commas
      | % %     nenums = length(separatorpos)+1 % number of enums is equal to number of commas + 1
      | % %     for i = 1:nenums,
      | % %         thisenum = char(enums(separatorpos(i):separatorpos(i+1)))
      | % %         
      | % %     end;
      | % end;
      | % set(gcbh,'MaskEnables',cbenables);
      | % % set(gcbh,'MaskValues',cbvalues);
      | % % try
      | % %     clear nenums possible_enums enumname enum_values dataportindices_enums cbvalues cbid cbenables i thisenum
      | % % catch
      | % % end
      mask Callback enum_class:
      | % if (enum_class == 'All'),
      | %     set_param(enum_vals,'Tunable','off')
      | % else
      | %     set_param(enum_vals,'Tunable','on')
      | % end;
      mask TypeOptions sel_indices: All | Specify indices
      mask Callback sel_indices:
      | % as of 10May2018, this block still has some issues with regards to
      | % populating the field with the enum values when the "All" radio button is
      | % selected and also setting the block values correctly.  It kind of works
      | % but is wonky.
      | 
      | cbid = get(gcbh); % get current block handle (in this case, is the mask)
      | cbvalues = cbid.MaskValues; % get the values from the mask;
      | cbenables = cbid.MaskEnables; % get the enables from the mask
      | if (ismember('All',cbvalues(2))), % if radio button selection (MaskValues = 2) is 'All'
      |     cbenables(3) = {'off'}; % disable the edit box
      |     [fpathstr,fnamestr,fextstr]=fileparts(char(cbvalues(4)));
      |     tenum_class = fnamestr; % assign value of enum name in textbox to variable
      |     enum_values = enumeration(tenum_class); % get enumeration values based on enum name in textbox
      |     nenums = length(enum_values); % # of enumeration values
      |     possible_enums = ['{' char(tenum_class) '.'];
      |     % get enum values and make cell
      |     for i = 1:nenums,
      |         thisenum = char(enum_values(i));
      |         if (i == 1),
      |             possible_enums = strcat(possible_enums,thisenum);
      |         else
      |             possible_enums = strcat(possible_enums,',',tenum_class,'.',thisenum);
      |         end;
      |     end;
      |     possible_enums = char(strcat(possible_enums,'}'));
      |     set(gcbh,'DataPortIndices',possible_enums);
      |     cbvalues(3) = cellstr(possible_enums);
      |     set(gcbh,'MaskEnables',cbenables);
      |     set(gcbh,'MaskValues',cbvalues);
      | else % if radio button selection (MaskValues = 2) is NOT 'All'
      |     cbenables(3) = {'on'}; % enable the edit box
      | end;
      | set(gcbh,'MaskEnables',cbenables);
      mask TypeOptions DataPortIndices: DataPortIndices
      mask DialogControl Container3 Prompt: Block parameters
      mask DialogControl DataPortIndices Prompt: Data port indices (e.g. {1,[2,3]}):
      mask DialogControl Container7 Prompt: Edit
      mask DialogControl Control2 Prompt: Browse...
      mask DialogControl Control2 Callback:
      | % who
      | % debug=1;
      | % if (debug), disp('browse'); end;
      | cbid = get(gcbh); % get current block handle (in this case, is the mask)
      | cbenables = cbid.MaskEnables; % get the enables from the mask
      | cbvalues = cbid.MaskValues; % get the values from the mask;
      | [fpathstr,fnamestr,fextstr]=fileparts(char(cbvalues(4)));
      | enum_class = fnamestr; % enum name
      | % enum_class = char(cbvalues(1));
      | enum_location = which(enum_class);
      | [fpathstr,fname,fext] = fileparts(enum_location);
      | enum_location = enum_location(1,:); % to prevent shadowed files
      | if (length(enum_location) == 0),
      |     [newfname,newfpathstr] = uigetfile; % file not found, ask user to select one
      | else
      |     [newfname,newfpathstr] = uigetfile(fpathstr);
      | end;
      | new_enum_location = fullfile(newfpathstr,newfname);
      | fileexists = 0;
      | try
      |     if (exist(new_enum_location) == 2), fileexists = 1; end;
      | catch
      | end;
      | if (fileexists),
      |     [fpathstr,fnamestr,fextstr]=fileparts(char(cbvalues(4)));
      |     %     cbvalues(1) = cellstr(newfname);
      |     cbvalues(1) = cellstr(fnamestr);
      |     cbvalues(2) = cellstr('All');
      |     cbvalues(4) = cellstr(new_enum_location);
      |     set(gcbh,'MaskValues',cbvalues);
      | end;
      | % if (debug), disp('browse end'); end;
      | % [fpath,fname,fext]=fileparts(new_enum_location);
      | cbenables(3) = {'off'}; % disable the edit box
      | [fpathstr,fnamestr,fextstr]=fileparts(char(cbvalues(4)));
      | tenum_class = fnamestr; % assign value of enum name in textbox to variable
      | enum_values = enumeration(tenum_class); % get enumeration values based on enum name in textbox
      | nenums = length(enum_values); % # of enumeration values
      | possible_enums = ['{' char(tenum_class) '.'];
      | % get enum values and make cell
      | for i = 1:nenums,
      |     thisenum = char(enum_values(i));
      |     if (i == 1),
      |         possible_enums = strcat(possible_enums,thisenum);
      |     else
      |         possible_enums = strcat(possible_enums,',',tenum_class,'.',thisenum);
      |     end;
      | end;
      | possible_enums = char(strcat(possible_enums,'}'));
      | set(gcbh,'DataPortIndices',possible_enums);
      | cbvalues(3) = cellstr(possible_enums);
      | set(gcbh,'MaskEnables',cbenables);
      | set(gcbh,'MaskValues',cbvalues);
      mask DialogControl Control3 Prompt: Edit
      mask DialogControl Control3 Callback:
      | cbid = get(gcbh); % get current block handle (in this case, is the mask)
      | cbvalues = cbid.MaskValues; % get the values from the mask;
      | fpath = char(cbvalues(4));
      | [fpathstr,fnamestr,fextstr] = fileparts(fpath);
      | if (exist(fpath) ~= 2),
      |     fline{1} =['classdef ' fnamestr ' < Simulink.IntEnumType'];
      |     fline{2} ='    enumeration';
      |     fline{3} ='        ENUM_ZERO(0)';
      |     fline{4} ='        ENUM_ONE(1)';
      |     fline{5} ='        ENUM_TWO(2)';
      |     fline{6} ='        ENUM_THREE(3)';
      |     fline{7} ='    end';
      |     fline{8} ='    methods (Static = true)';
      |     fline{9} ='    end';
      |     fline{10}='end';
      |     fid = fopen(fpath,'w');
      |     for i = 1:length(fline),
      |         fprintf(fid,fline{i});
      |         fprintf(fid,'\n');
      |     end;
      |     fclose(fid);
      | end;
      | edit(fpath);
      mask Display: port_label('input', 1, ['                ' enum_class]);
  If_Then_Else : Subsystem  TreatAsAtomicUnit=on  mask(If-then-else (EmE)){}
      mask help: Passes through the "then" port when "if" = TRUE, otherwise it passes through the "else" port.
      mask Display:
      | plot([0.25 0.82],[0.87 0.87])
      | plot([0.47 0.77 1],[0.2 0.5 0.5])
      | plot([0.82 0.82],[0.55 0.87])
      | plot([0.75 0.82 0.84 0.88],[0.6 0.55 0.55 0.6])
      | port_label('input',1,'If')
      | port_label('input',2,'Then')
      | port_label('input',3,'Else')
  Multiport Switch : MultiPortSwitch  DataPortForDefault=Additional data port  DiagnosticForDefault=None  InputSameDT=on
  Mux : Mux  Inputs=2

== system EmE_MBD_Blockset/Sinks ==
  Terminator : Terminator
  Out : Outport  OutputWhenDisabled=reset  InitialOutput=InitialOutput  mask(Outport (EmE)){Port=1, InitialOutput=[], OutputWhenDisabled=reset, SourceOfInitialOutputValue=Dialog}
      mask prompts: Port "Simulink:blkprm_prompts:InOutportPortNum"; InitialOutput "Simulink:blkprm_prompts:OutportInitOutput"; OutputWhenDisabled "Simulink:blkprm_prompts:OutportDisabledOutput"; SourceOfInitialOutputValue "Simulink:blkprm_prompts:OutportInitOutputSrc"
      mask help: Provide an output port for a subsystem or model. The 'Output when disabled' and 'Initial output' parameters only apply to conditionally executed subsystems. When a conditionally executed subsystem is disabled, the output is either held at its last value or set to the 'Initial output'.
      mask init:
      | anyenableports = ~isempty(find_system(get(gcbh,'Parent'),'BlockType','EnablePort'));
      | anytriggerports = ~isempty(find_system(get(gcbh,'Parent'),'BlockType','TriggerPort'));
      | if (or(anyenableports,anytriggerports)),
      |     set(gcbh,'AttributesFormatString','IC: %<InitialOutput>\nDisabled value: %<OutputWhenDisabled>')
      | else
      |     set(gcbh,'AttributesFormatString','')
      | end;
      | clear anyenableports anytriggerports
      settings: CopyFcn=|
      | try
      | pathofenableports = find_system(get(gcbh,'Parent'),'BlockType','EnablePort');
      | anyenableports_incurrentpath = getfullname(pathofenableports);
      | anyenableports_incurrentpath = char(anyenableports_incurrentpath{1});
      | anyenableports = strcmpi(get(gcbh,'Parent'),anyenableports_incurrentpath);
      | pathoftriggerports = find_system(get(gcbh,'Parent'),'BlockType','TriggerPort');
      | anytriggerports_incurrentpath = getfullname(pathoftriggerports);
      | anytriggerports_incurrentpath = char(anytriggerports_incurrentpath{1});
      | anytriggerports = strcmpi(get(gcbh,'Parent'),anytriggerports_incurrentpath);
      | if (or(anyenableports,anytriggerports)),
      | set(gcbh,'AttributesFormatString','IC: %<InitialOutput>\nDisabled value: %<OutputWhenDisabled>')
      | else
      | set(gcbh,'AttributesFormatString','')
      | end;
      | catch
      | end;
      | clear anyenableports anytriggerports pathofenableports pathoftriggerports
      settings: NameChangeFcn=|
      | try
      | pathofenableports = find_system(get(gcbh,'Parent'),'BlockType','EnablePort');
      | anyenableports_incurrentpath = getfullname(pathofenableports);
      | anyenableports_incurrentpath = char(anyenableports_incurrentpath{1});
      | anyenableports = strcmpi(get(gcbh,'Parent'),anyenableports_incurrentpath);
      | pathoftriggerports = find_system(get(gcbh,'Parent'),'BlockType','TriggerPort');
      | anytriggerports_incurrentpath = getfullname(pathoftriggerports);
      | anytriggerports_incurrentpath = char(anytriggerports_incurrentpath{1});
      | anytriggerports = strcmpi(get(gcbh,'Parent'),anytriggerports_incurrentpath);
      | if (or(anyenableports,anytriggerports)),
      | set(gcbh,'AttributesFormatString','IC: %<InitialOutput>\nDisabled value: %<OutputWhenDisabled>')
      | else
      | set(gcbh,'AttributesFormatString','')
      | end;
      | catch
      | end;
      | clear anyenableports anytriggerports pathofenableports pathoftriggerports
      settings: MoveFcn=|
      | try
      | pathofenableports = find_system(get(gcbh,'Parent'),'BlockType','EnablePort');
      | anyenableports_incurrentpath = getfullname(pathofenableports);
      | anyenableports_incurrentpath = char(anyenableports_incurrentpath{1});
      | anyenableports = strcmpi(get(gcbh,'Parent'),anyenableports_incurrentpath);
      | pathoftriggerports = find_system(get(gcbh,'Parent'),'BlockType','TriggerPort');
      | anytriggerports_incurrentpath = getfullname(pathoftriggerports);
      | anytriggerports_incurrentpath = char(anytriggerports_incurrentpath{1});
      | anytriggerports = strcmpi(get(gcbh,'Parent'),anytriggerports_incurrentpath);
      | if (or(anyenableports,anytriggerports)),
      | set(gcbh,'AttributesFormatString','IC: %<InitialOutput>\nDisabled value: %<OutputWhenDisabled>')
      | else
      | set(gcbh,'AttributesFormatString','')
      | end;
      | catch
      | end;
      | clear anyenableports anytriggerports pathofenableports pathoftriggerports
      mask TypeOptions Port: Port
      mask TypeOptions InitialOutput: InitialOutput
      mask TypeOptions OutputWhenDisabled: OutputWhenDisabled
      mask TypeOptions SourceOfInitialOutputValue: SourceOfInitialOutputValue
      mask DialogControl Port Prompt: Port number:
      mask DialogControl InitialOutput Prompt: Initial output:
      mask DialogControl OutputWhenDisabled Prompt: Output when disabled:
      mask DialogControl SourceOfInitialOutputValue Prompt: Source of initial output value:
